simulink model "selector_test"  (Simulink 8.4)
settings: Solver=VariableStepDiscrete  StartTime=0.0  StopTime=0  MaxStep=1  RelTol=1e-3
settings Model: Creator=arnaud  LastModifiedBy=arnaud
settings DataIOCC: ExternalInput=xin  SaveFormat=Structure

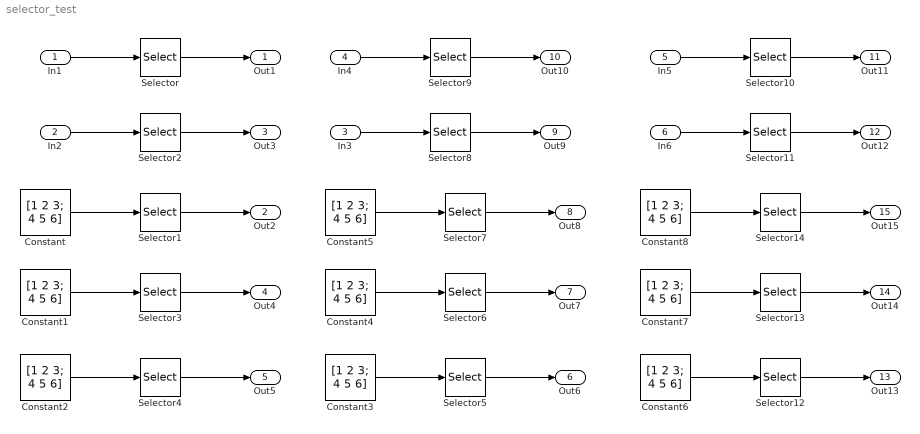
== system selector_test ==
  In1 : Inport  PortDimensions=3
  In2 : Inport  Port=2  PortDimensions=3
  In3 : Inport  Port=3  PortDimensions=3
  In4 : Inport  Port=4  PortDimensions=3
  In5 : Inport  Port=5  PortDimensions=3
  In6 : Inport  Port=6  PortDimensions=3
  Constant{,1..8} (9 alike) : Constant  Value=[1 2 3; 4 5 6]
  Selector : Selector  IndexMode=Zero-based  InputPortWidth=3  Indices=[1 0 0]
  Selector1 : Selector  NumberOfDimensions=2  InputPortWidth=3  IndexOptions=Index vector (dialog),Index vector (dialog)  Indices=[2 1],1  OutputSizes=1,2
  Selector10 : Selector  InputPortWidth=3  IndexOptions=Starting index (dialog)
  Selector11 : Selector  InputPortWidth=3  IndexOptions=Starting index (dialog)  OutputSizes=2
  Selector12 : Selector  NumberOfDimensions=2  InputPortWidth=3  IndexOptions=Starting index (dialog),Select all  Indices=1,1  OutputSizes=1,2
  Selector13 : Selector  NumberOfDimensions=2  InputPortWidth=3  IndexOptions=Index vector (dialog),Starting index (dialog)  Indices=[2 1],1  OutputSizes=1,2
  Selector14 : Selector  NumberOfDimensions=2  IndexMode=Zero-based  InputPortWidth=3  IndexOptions=Index vector (dialog),Starting index (dialog)  Indices=[1 0],0  OutputSizes=1,2
  Selector2 : Selector  InputPortWidth=3  Indices=2
  Selector3 : Selector  NumberOfDimensions=2  IndexMode=Zero-based  InputPortWidth=3  IndexOptions=Index vector (dialog),Select all  Indices=[1 0],1  OutputSizes=1,2
  Selector4 : Selector  NumberOfDimensions=2  IndexMode=Zero-based  InputPortWidth=3  IndexOptions=Select all,Select all  Indices=0,1  OutputSizes=1,2
  Selector5 : Selector  NumberOfDimensions=2  InputPortWidth=3  IndexOptions=Select all,Select all  Indices=0,1  OutputSizes=1,2
  Selector6 : Selector  NumberOfDimensions=2  InputPortWidth=3  IndexOptions=Index vector (dialog),Select all  Indices=[2 1],1  OutputSizes=1,2
  Selector7 : Selector  NumberOfDimensions=2  IndexMode=Zero-based  InputPortWidth=3  IndexOptions=Index vector (dialog),Index vector (dialog)  Indices=[1 0],0  OutputSizes=1,2
  Selector8 : Selector  IndexMode=Zero-based  InputPortWidth=3
  Selector9 : Selector  InputPortWidth=3  Indices=[2 1 1]
  Out1 : Outport
  Out2 : Outport  Port=2
  Out3 : Outport  Port=3
  Out4 : Outport  Port=4
  Out5 : Outport  Port=5
  Out6 : Outport  Port=6
  Out7 : Outport  Port=7
  Out8 : Outport  Port=8
  Out9 : Outport  Port=9
  Out10 : Outport  Port=10
  Out11 : Outport  Port=11
  Out12 : Outport  Port=12
  Out13 : Outport  Port=13
  Out14 : Outport  Port=14
  Out15 : Outport  Port=15
  wires:
  Selector/1 -> Out1/1
  In1/1 -> Selector/1
  Selector1/1 -> Out2/1
  Constant/1 -> Selector1/1
  Selector2/1 -> Out3/1
  In2/1 -> Selector2/1
  Selector3/1 -> Out4/1
  Constant1/1 -> Selector3/1
  Selector4/1 -> Out5/1
  Constant2/1 -> Selector4/1
  Selector5/1 -> Out6/1
  Constant3/1 -> Selector5/1
  Selector6/1 -> Out7/1
  Constant4/1 -> Selector6/1
  Selector7/1 -> Out8/1
  Constant5/1 -> Selector7/1
  Selector8/1 -> Out9/1
  In3/1 -> Selector8/1
  Selector9/1 -> Out10/1
  In4/1 -> Selector9/1
  Selector10/1 -> Out11/1
  In5/1 -> Selector10/1
  Selector11/1 -> Out12/1
  In6/1 -> Selector11/1
  Selector12/1 -> Out13/1
  Constant6/1 -> Selector12/1
  Selector13/1 -> Out14/1
  Constant7/1 -> Selector13/1
  Selector14/1 -> Out15/1
  Constant8/1 -> Selector14/1
